simulink subsystem "ControladorMotores"  (R2023b)
settings: Solver=VariableStepAuto  StartTime=0.0  StopTime=10.0  RelTol=1e-3
settings Model: Creator=Enrique  LastModifiedBy=Enrique

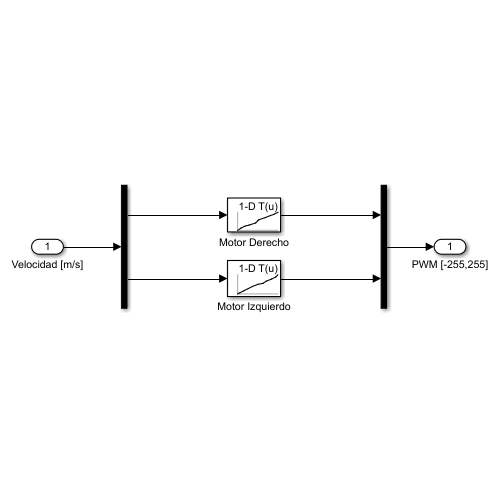
[thumbnail: Simulink's stored preview of the top-level diagram]
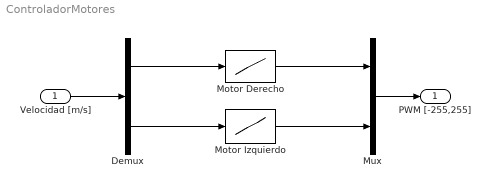
== system ControladorMotores ==
  Velocidad [m/s] : Inport
  Demux : Demux  Outputs=2
  Motor Derecho : Lookup_n-D  NumberOfTableDimensions=1  BreakpointsForDimension1=[-0.394065856933594 -0.328388214111328 -0.25177001953125 -0.153251647949219 -0.0437850952148438 0 0.0328389555215836 0.153248310089111 0.251765251159668 0.328390121459961 0.394069671630859]  Table=[-255 -200 -150 -100 -50 0 50 100 150 200 255]  InternalRulePriority=Speed  RndMeth=Simplest
  Motor Izquierdo : Lookup_n-D  NumberOfTableDimensions=1  BreakpointsForDimension1=[-0.440517425537109 -0.38255500793457 -0.301408767700195 -0.208666324615479 -0.115925908088684 0 0.115928649902344 0.197074890136719 0.301406860351563 0.382553100585938 0.428928375244141]  Table=[-255 -200 -150 -100 -50 0 50 100 150 200 255]  InternalRulePriority=Speed  RndMeth=Simplest
  Mux : Mux  Inputs=2
  PWM [-255,255] : Outport
  wires:
  Velocidad [m/s]/1 -> Demux/1
  Mux/1 -> PWM [-255,255]/1
  Demux/2 -> Motor Izquierdo/1
  Motor Izquierdo/1 -> Mux/2
  Demux/1 -> Motor Derecho/1
  Motor Derecho/1 -> Mux/1
